simulink model "pendulumSimA"  (R2018a)
settings: Solver=VariableStepAuto  StartTime=0.0  StopTime=100  RelTol=1e-3
InitFcn:
  | params
undefined symbols (not defined in the file or in its folder): P
settings Model: Creator=mark  LastModifiedBy=mark

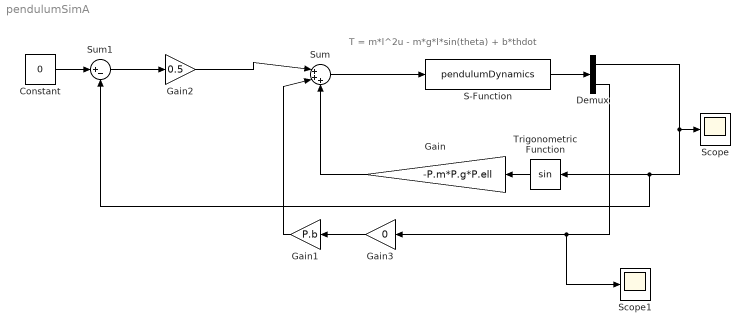
== system pendulumSimA ==
  note: T = m*l^2u - m*g*l*sin(theta) + b*thdot
  Constant : Constant  Value=0
  Demux : Demux  Outputs=2
  Gain : Gain  Gain=-P.m*P.g*P.ell
  Gain1 : Gain  Gain=P.b
  Gain2 : Gain  Gain=0.5
  Gain3 : Gain  Gain=0
  S-Function : S-Function  FunctionName=pendulumDynamics  Parameters=P  SFunctionDeploymentMode=off  EnableBusSupport=off
  Scope : Scope
  Scope1 : Scope
  Sum : Sum  Inputs=|+++
  Sum1 : Sum  Inputs=|+-
  Trigonometric Function : Trigonometry
  wires:
  S-Function/1 -> Demux/1
  Demux/1 -> Scope/1, Sum1/2, Trigonometric Function/1
  Trigonometric Function/1 -> Gain/1
  Demux/2 -> Scope1/1, Gain3/1
  Gain/1 -> Sum/3
  Gain1/1 -> Sum/2
  Sum1/1 -> Gain2/1
  Gain2/1 -> Sum/1
  Constant/1 -> Sum1/1
  Sum/1 -> S-Function/1
  Gain3/1 -> Gain1/1
